simulink subsystem "Prova_1"  (R2024b)
settings: Solver=VariableStepAuto  StartTime=0.0  StopTime=10.0  RelTol=1e-3
settings Model: Creator=sabpi  LastModifiedBy=sabpi

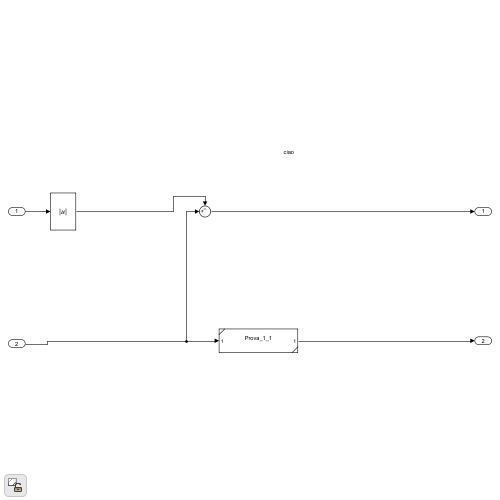
[thumbnail: Simulink's stored preview of the top-level diagram]
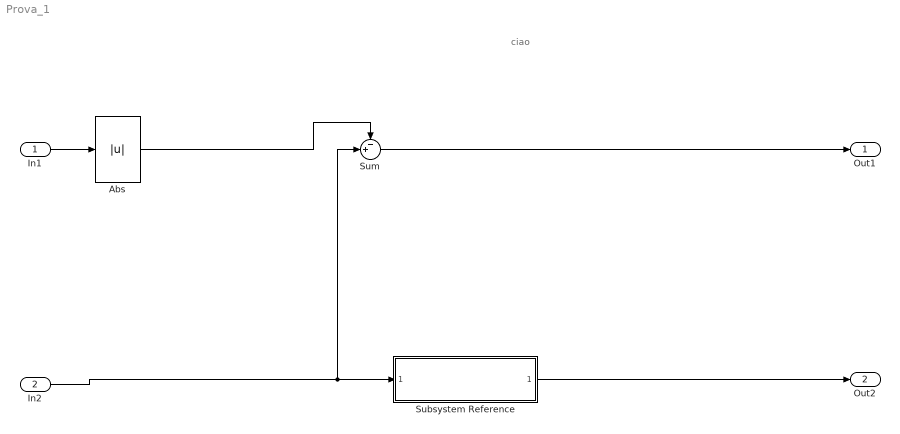
== system Prova_1 ==
  note: ciao
  In1 : Inport
  In2 : Inport  Port=2
  Abs : Abs  SaturateOnIntegerOverflow=off
  Subsystem Reference : Subsystem  ReferencedSubsystem=Prova_1_1
  Sum : Sum  Inputs=-+|
  Out1 : Outport
  Out2 : Outport  Port=2
  wires:
  Sum/1 -> Out1/1
  In1/1 -> Abs/1
  In2/1 -> Sum/2, Subsystem Reference/1
  Subsystem Reference/1 -> Out2/1
  Abs/1 -> Sum/1
